simulink model "MVB4Single"  (R2013b)
settings: Solver=FixedStepDiscrete  SolverMode=SingleTasking  StartTime=0  StopTime=8000  RelTol=1e-3
model workspace (MAT data in the model file):
  logicAddr = 2
settings Model: Creator=qiji  LastModifiedBy=qiji
settings DataIOCC: SignalLoggingSaveFormat=ModelDataLogs
settings OptimizationCC: BlockReduction=off  ConditionallyExecuteInputs=off  InlineParams=on
settings DebuggingCC: UnderspecifiedInitializationDetection=Simplified  MultiTaskDSMMsg=warning  MultiTaskCondExecSysMsg=none  SingleTaskRateTransMsg=error  SFUnusedDataAndEventsDiag=none
settings RTWCC: IncludeERTFirstTime=on
settings GRTTargetCC: CodeReplacementLibrary=None  CPPClassGenCompliant=on
settings ConfigurationSet: Description=SimMechanics 2G

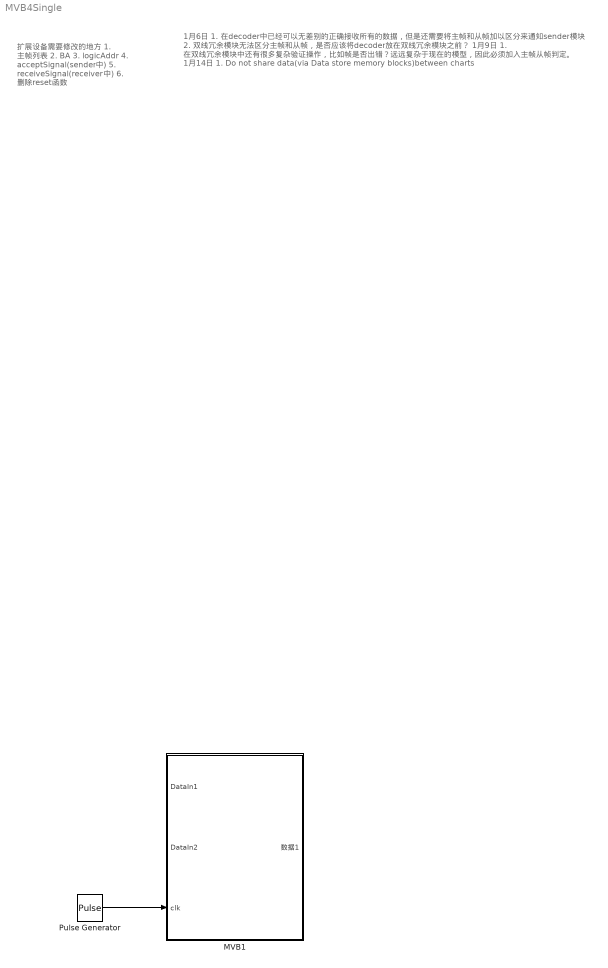
== system MVB4Single ==
  note: 扩展设备需要修改的地方
      | 1. 主帧列表
      | 2. BA
      | 3. logicAddr
      | 4. acceptSignal(sender中)
      | 5. receiveSignal(receiver中)
      | 6. 删除reset函数
  note: 1月6日
      | 1. 在decoder中已经可以无差别的正确接收所有的数据，但是还需要将主帧和从帧加以区分来通知sender模块
      | 2. 双线冗余模块无法区分主帧和从帧，是否应该将decoder放在双线冗余模块之前？
      | 1月9日
      | 1. 在双线冗余模块中还有很多复杂验证操作，比如帧是否出错？远远复杂于现在的模型，因此必须加入主帧从帧判定。
      | 1月14日
      | 1. Do not share data(via Data store memory blocks)between charts
  MVB1 : Subsystem
  Pulse Generator : DiscretePulseGenerator  Amplitude=true
  wires:
  Pulse Generator/1 -> MVB1/3("clk ")

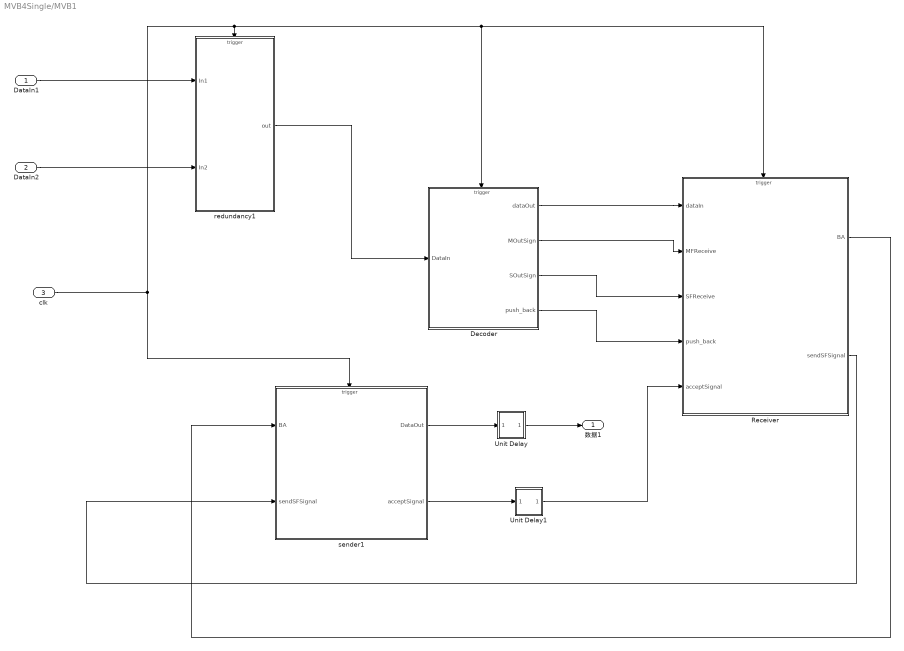
== system MVB4Single/MVB1 ==
  DataIn1 : Inport
  DataIn2 : Inport  Port=2
  "clk " : Inport  Port=3
  Decoder : Stateflow chart  TreatAsAtomicUnit=on
  Receiver : Stateflow chart  TreatAsAtomicUnit=on
  Unit Delay : Subsystem
  Unit Delay1 : Subsystem
  redundancy1 : Stateflow chart  TreatAsAtomicUnit=on
  sender1 : Stateflow chart  TreatAsAtomicUnit=on
  数据1 : Outport
  wires:
  DataIn1/1 -> redundancy1/1(In1)
  DataIn2/1 -> redundancy1/2(In2)
  redundancy1/1(out) -> Decoder/1(DataIn)
  Unit Delay/1(Out) -> 数据1/1
  "clk "/1 -> Decoder/Trigger, Receiver/Trigger, redundancy1/Trigger, sender1/Trigger
  Decoder/1(dataOut) -> Receiver/1(dataIn)
  Decoder/2(MOutSign) -> Receiver/2(MFReceive)
  Decoder/3(SOutSign) -> Receiver/3(SFReceive)
  Decoder/4(push_back) -> Receiver/4(push_back)
  Receiver/1(BA) -> sender1/1(BA)
  Unit Delay1/1(Out) -> Receiver/5(acceptSignal)
  Receiver/2(sendSFSignal) -> sender1/2(sendSFSignal)
  sender1/1(DataOut) -> Unit Delay/1(In1)
  sender1/2(acceptSignal) -> Unit Delay1/1(In1)

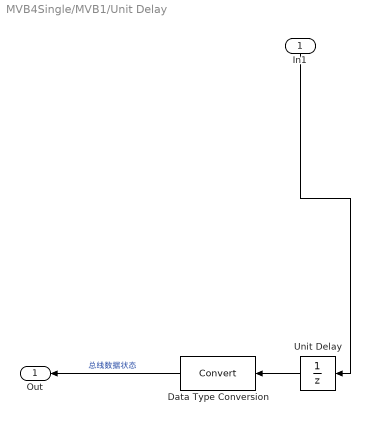
== system MVB4Single/MVB1/Unit Delay ==
  In1 : Inport
  Data Type Conversion : DataTypeConversion
  Unit Delay : UnitDelay  SampleTime=-1
  Out : Outport
  wires:
  In1/1 -> Unit Delay/1
  Unit Delay/1 -> Data Type Conversion/1
  Data Type Conversion/1 -> Out/1  "总线数据状态"

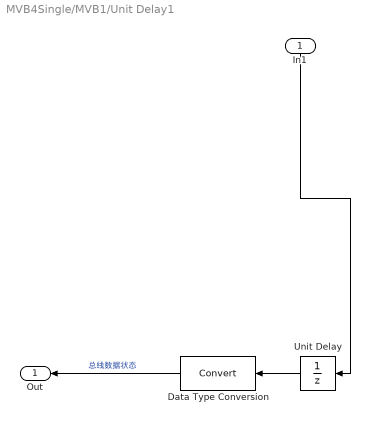
== system MVB4Single/MVB1/Unit Delay1 ==
  In1 : Inport
  Data Type Conversion : DataTypeConversion
  Unit Delay : UnitDelay  SampleTime=-1
  Out : Outport
  wires:
  Data Type Conversion/1 -> Out/1  "总线数据状态"
  Unit Delay/1 -> Data Type Conversion/1
  In1/1 -> Unit Delay/1

== stateflow chart MVB4Single/MVB1/redundancy1 ==
  settings: executeAtInitialization=1  initializeOutput=1
  state sign_maker [parallel]
    settings: executionOrder=1
    state sign1 [parallel]
      settings: executionOrder=1
      state trans
        sign_maker.sign1.trans -> sign_maker.sign1.trans [order 1] : CLK
            | {
            | buffer = bitoperate.shiftbit(buffer, 1) + In1;
            | count++;
            | }
      state none
        en:
        count=2;
        buffer=1;
      state judge
      (default) -> sign_maker.sign1.none : {count=0;buffer=0;}
      sign_maker.sign1.none -> sign_maker.sign1.trans : [In1==1]{sign1 = true;}
      sign_maker.sign1.judge -> sign_maker.sign1.trans [order 2] : {buffer=0;count=0;}
      sign_maker.sign1.judge -> sign_maker.sign1.none [order 1] : [judgeEnd(buffer)]
          | {sign1 = false;}
      sign_maker.sign1.trans -> sign_maker.sign1.judge [order 1] : [count==32]
          | {buffer=ManchesterDecoding(buffer);
          | }
    state sign2 [parallel]
      settings: executionOrder=2
      state trans
        sign_maker.sign2.trans -> sign_maker.sign2.trans [order 1] : CLK
            | {
            | buffer = bitoperate.shiftbit(buffer, 1) + In2;
            | count++;
            | }
      state none
        en:
        count=2;
        buffer=1;
      state judge
      (default) -> sign_maker.sign2.none : {count=0;buffer=0;}
      sign_maker.sign2.none -> sign_maker.sign2.trans : [In2==1]{sign2 = true;}
      sign_maker.sign2.judge -> sign_maker.sign2.trans [order 2] : {buffer=0;count=0;}
      sign_maker.sign2.judge -> sign_maker.sign2.none [order 1] : [judgeEnd(buffer)]
          | {sign2 = false;}
      sign_maker.sign2.trans -> sign_maker.sign2.judge [order 1] : [count==32]
          | {buffer=ManchesterDecoding(buffer);
          | }
  state bitoperate [group]
  note: 从上一个接收事件后总线寂静1.4ms则产生一总线寂静的通知
  state Timer1 [parallel]
    settings: executionOrder=2
    state Timer
    state start
    state TimeOut
      entry:
      trust = false;
    start -> Timer : [judge(sign1, sign2, trust) == false]
    (default) -> start
    Timer -> start [order 1] : [judge(sign1, sign2,  trust) == true]
    TimeOut -> start
    Timer -> TimeOut [order 2] : [after(140, CLK) && judge(sign1, sign2,  trust) == false]
  note: 上一个主帧接收后1.3ms没有收到主帧产生一个主帧超时的通知。
  note: 收到主帧后42.7us没有收到从帧产生从帧超时的通知。
  note: 信任线未收到数据，而观察线收到数据时切换
  state observer [parallel]
    settings: executionOrder=3
    state A
      entry:
      trust = true;
    state B
      entry:
      trust = false;
    observer.A -> observer.B : [judge(sign1, sign2, trust) == false]
    (default) -> observer.A
    observer.B -> observer.A : [judge(sign1, sign2, trust) == false]
  state trans [parallel]
    settings: executionOrder=4
    state A
      during:
      out = In1;
    state B
      during:
      out = In2;
    trans.A -> trans.B : [trust == false]{out = In2;}
    (default) -> trans.A
    trans.B -> trans.A : [trust == true]{out = In1;}
  data: r function_output boolean; data function_input uint16; buffer local uint32; count local uint32; buffer local uint32; count local uint32; r function_output uint32; data function_input uint32; num function_input uint32; r function_output uint32; data function_input uint32; num function_input uint32; r function_output uint32; r function_output boolean; dataIn1 function_input uint32; dataIn2 function_input uint32; t function_input boolean; r function_output boolean; dataIn1 function_input boolean; dataIn2 function_input boolean; t function_input boolean; In1 input uint32; In2 input uint32; out output uint32; trust local boolean =true; sign1 local boolean; sign2 local boolean
  events: CLK input RISING_EDGE_EVENT
  function r = judgeEnd(data):
    | function r = judgeEnd(data)
    | bit1 = bitget(data, 1);
    | bit2 = bitget(data, 2);
    | bit3 = bitget(data, 3);
    | bit4 = bitget(data, 4);
    | if bit1==1 && bit2==1 && bit3==0 && bit4==0
    |     r = true;
    | else
    |     r = false;
    | end
  function r = ManchesterDecoding(data):
    | function r = ManchesterDecoding(data)
    | r = uint32(0);
    | for i = (1:2:32)
    |     x0 = bitget(data, i);
    |     x1 = bitget(data, i+1);
    |     if x0==0 && x1==1
    |         r = bitset(r, (i+1)/2, 1);
    |     else
    |         r = bitset(r, (i+1)/2, 0);
    |     end
    | end
  function r = getbit(num):
    | function r = getbit(num)
    | r = bitget(num, 32);
  function r = shiftbit(data, num):
    | function r = shiftbit(data, num)
    | r = bitshift(data, num);
    | %for i=1:cnt
    | %   r = bitset(r, i, 0);
    | %end
  function r = judge(dataIn1, dataIn2, t):
    | function r = judge(dataIn1, dataIn2, t)
    | r = true;
    | if t == true
    |     if dataIn1==false
    |         r = false;
    |     end
    | else
    |     if dataIn2==false
    |         r = false;
    |     end
    | end
  function r = judge( dataIn1, dataIn2, t):
    | function r = judge( dataIn1, dataIn2, t)
    | r = true;
    | % 如果数据线1没有收到数据而数据线2收到了
    | if t == true
    |     if dataIn1==false && dataIn2==true
    |         r = false;
    |     end
    | else
    |     if dataIn2==false && dataIn1==true
    |         r = false;
    |     end
    | end

== stateflow chart MVB4Single/MVB1/sender1 ==
  settings: executeAtInitialization=1  initializeOutput=1
  state SFSender [parallel]
    settings: executionOrder=1
    note: send**Signd的置位在接收到了请求数据的主帧后置位
    state sender [parallel]
      settings: executionOrder=1
      state wait
      state sendRandomSF
      state sendOK
      state sendInfo
      state transmission
        en:
        enterTrans = true;
        ex:
        enterTrans = false;
      (default) -> SFSender.sender.wait
      SFSender.sender.wait -> sendRandomSF [order 1] : [sendSFSignal==1]
      SFSender.sender.wait -> sendInfo [order 3] : [ sendSFSignal==2]
      SFSender.sender.wait -> sendOK [order 2] : [sendSFSignal==3]
      sendRandomSF -> SFSender.sender.transmission : {SFIndex = uint8(0);}
      sendOK -> SFSender.sender.transmission : {SFIndex = uint8(2);
          | init();
          | }
      sendInfo -> SFSender.sender.transmission : {SFIndex = uint8(1);}
      SFSender.sender.transmission -> SFSender.sender : [SFTransDone == true]
          | {DataOut = uint32(0);}
          | /{SFTransDone = false;}
    state sendHolder [parallel]
      settings: executionOrder=2
      state judge
      state full
        SFSender.sendHolder.full -> SFSender.sendHolder.full [order 1] : CLK
            | {
            | DataOut = bitoperate.getbit(input);
            | input = bitoperate.shiftbit(input, uint32(1));
            | count = count + uint8(1);
            | }
      state empty
      SFSender.sendHolder.judge -> SFSender.sendHolder.empty [order 2] : {
          | SFCurrentIndex = uint8(2);
          | SFTransDone = true;
          | }
      SFSender.sendHolder.full -> SFSender.sendHolder.judge [order 1] : [count == uint8(32)]
          | {
          | SFCurrentIndex = SFCurrentIndex + uint8(1);
          | }
      SFSender.sendHolder.judge -> SFSender.sendHolder.full [order 1] : [SFCurrentIndex <= SFT[SFIndex*16 + 1]]
          | {
          | input = ManchesterEncoding(uint32(SFT[SFIndex*16+SFCurrentIndex]));
          | count = uint8(0);
          | }
      (default) -> SFSender.sendHolder.empty : {
          | SFCurrentIndex = uint8(2);
          | SFTransDone = false;
          | }
      SFSender.sendHolder.empty -> SFSender.sendHolder.full : [enterTrans == true]
          | {
          | input = ManchesterEncoding(uint32(SFT[SFIndex*16+SFCurrentIndex]));
          | DataOut = uint32(0);
          | count = uint8(0);
          | }
  state MFSender [parallel]
    settings: executionOrder=2
    state sender [parallel]
      settings: executionOrder=2
      state transmission
        en:
        enterTrans = true;
        acceptSignal =setAcceptSignal(MFT[MFIndex*16+3]);
        ex:
        enterTrans = false;
      state sleep
      state wait
      (default) -> sleep : {
          | init();
          | }
      MFSender.sender.transmission -> sleep : [MFTransDone==true]
          | {
          | DataOut = uint32(0);
          | MFIndex = MFIndex + uint8(1);
          | MFTransDone=false;
          | }
      sleep -> MFSender.sender.wait : every(150, CLK)
          | [master==true]
      MFSender.sender.wait -> MFSender.sender.transmission
    state sendHolder [parallel]
      settings: executionOrder=3
      state judge
      state full
        MFSender.sendHolder.full -> MFSender.sendHolder.full [order 1] : CLK
            | {
            | DataOut = bitoperate.getbit(input);
            | input = bitoperate.shiftbit(input, uint32(1));
            | count = count + uint8(1);
            | }
      state empty
      MFSender.sendHolder.judge -> MFSender.sendHolder.empty [order 2] : {
          | MFCurrentIndex = uint8(2);
          | MFTransDone=true;
          | }
      MFSender.sendHolder.full -> MFSender.sendHolder.judge [order 1] : [count == uint8(32)]
          | {
          | MFCurrentIndex = MFCurrentIndex + uint8(1);
          | }
      MFSender.sendHolder.judge -> MFSender.sendHolder.full [order 1] : [MFCurrentIndex <= MFT[MFIndex*16 + 1]]
          | {
          | input =ManchesterEncoding(uint32(MFT[MFIndex*16+MFCurrentIndex]));
          | count = uint8(0);
          | }
      (default) -> MFSender.sendHolder.empty : {
          | MFCurrentIndex = uint8(2);
          | MFTransDone=false;
          | }
      MFSender.sendHolder.empty -> MFSender.sendHolder.full : [enterTrans == true]
          | {
          | input = ManchesterEncoding(uint32(MFT[MFIndex*16+MFCurrentIndex]));
          | DataOut = uint32(0);
          | count = uint8(0);
          | }
    state BAHolder [parallel]
      settings: executionOrder=1
      state false
        du:
        master = false;
      state true
        du:
        master = true;
      false -> true : [BA == true]
          | {master = true;}
      (default) -> true
      true -> false : [BA == true]
          | {master =false;}
  state init [function]
    note: F_code=0
        | addr=2
        | 0010//1100/0111/0001
        | 0101//0000/0000/0000
        | 0010//1010/1000/1110
        | 0000/0000/0011//0011
        | F_code=8
        | addr=2
        | 0010//1100/0111/0001
        | 0101//1000/0000/0000
        | 0010//1010/1000/1110
        | 0000/0000/0011//0011
        | F_code=0
        | addr=2
        | 0010//1100/0111/0001
        | 0101//1111/0000/0000
        | 0010//1010/1000/1110
        | 0000/0000/0011//0011
    note: 请求随机从帧
        | 请求随机从帧
        | 请求2号的信息
        | 请求转移到2号
    note: SFT(1)代表随机的从帧
        | SFT(2)代表回复接受主权
        | SFT(3)代表回复设备ACT和BA
    (default) -> (junction 77) : {
        | MFIndex = uint8(0);
        | acceptSignal = uint8(0);
        | MFT[1] = uint16(5);
        | MFT[2] = uint16(11377);
        | MFT[3] = uint16(20480);
        | MFT[4] = uint16(10894);
        | MFT[5] = uint16(51);
        |
        | MFT[17] = uint16(5);
        | MFT[18] = uint16(11377);
        | MFT[19] = uint16(20480);
        | MFT[20] = uint16(14990);
        | MFT[21] = uint16(51);
        |
        | MFT[33] = uint16(5);
        | MFT[34] = uint16(11377);
        | MFT[35] = uint16(22528);
        | MFT[36] = uint16(10894);
        | MFT[37] = uint16(51);
        |
        | MFT[49] = uint16(5);
        | MFT[50] = uint16(11377);
        | MFT[51] = uint16(24320);
        | MFT[52] = uint16(10894);
        | MFT[53] = uint16(51);
        |
        |
        | SFT[1] = uint16(4);
        | SFT[2] = uint16(10894);
        | SFT[3] = uint16(12428);
        | SFT[4] = uint16(19);
        | SFT[17] = uint16(4);
        | SFT[18] = uint16(10894);
        | SFT[19] = uint16(12832);
        | SFT[20] = uint16(3);
        | SFT[33] = uint16(4);
        | SFT[34] = uint16(10894);
        | SFT[35] = uint16(14464);
        | SFT[36] = uint16(3);
        | }
  state bitoperate [group]
  note: MFT(1) = 5;
      | MFT(2) = 11377;
      | MFT(3) = 20480;
      | MFT(4) = 10894;
      | MFT(5) = 51;
      |
      | MFT(17) = 5;
      | MFT(18) = 11377;
      | MFT(19) = 20480;
      | MFT(20) = 10894;
      | MFT(21) = 51;
      |
      | MFT(33) = 5;
      | MFT(34) = 11377;
      | MFT(35) = 22528;
      | MFT(36) = 10894;
      | MFT(37) = 51;
      |
      | MFT(49) = 5
      | MFT(50) = 11377;
      | MFT(52) = 24320;
      | MFT(53) = 10894;
      | MFT(54) = 51;
  data: SFCurrentIndex local uint8; count local uint8; input local uint32; SFTransDone local boolean; SFIndex local uint8; enterTrans local boolean; data function_input uint16; Signal function_output uint8; bit1 temporary uint16; bit2 temporary uint16; bit3 temporary uint16; bit0 temporary uint16; i function_input double; r function_output uint8; MFCurrentIndex local uint8; count local uint8; input local uint32; MFTransDone local boolean; enterTrans local boolean; data function_input uint32; r function_output uint32; r function_output uint32; data function_input uint32; num function_input uint32; r function_output uint32; data function_input uint32; num function_input uint32; r function_output uint32; BA input boolean; sendSFSignal input uint8; MFT local uint16 size=100; SFT local uint16 size=100; DataOut output uint32; acceptSignal output uint8; MFIndex local uint8; master local boolean
  events: CLK input RISING_EDGE_EVENT
  function Signal = setAcceptSignal(data):
    | function Signal = setAcceptSignal(data)
    | bit0 = uint16(bitget(data, 9));
    | bit1 = uint16(bitget(data, 10));
    | bit2 = uint16(bitget(data, 11));
    | bit3 = uint16(bitget(data, 12));
    | fcode = bit0+bit1*2+bit2*4+bit3*8;
    | Signal=uint8(0);
    | if fcode==0
    |     Signal=uint8(1);
    | elseif fcode==8
    |     Signal=uint8(2);
    | elseif fcode==15
    |     Signal=uint8(3);
    | end
  function r = reset(i):
    | function r = reset(i)
    | if i==2
    |     r = uint8(0);
    | else
    |     r = uint8(i);
    | end
  function r = ManchesterEncoding(data):
    | function r = ManchesterEncoding(data)
    | r = data;
    | for i = 1:16
    |     x = bitget(data, i);
    |     if x == 0
    |         r = bitset(r, i*2-1, 1);
    |         r = bitset(r, i*2, 0);
    |     else
    |         r = bitset(r, i*2-1, 0);
    |         r = bitset(r, i*2, 1);
    |     end
    | end
  function r = ManchesterDecoding(data):
    | function r = ManchesterDecoding(data)
    | r = uint32(0);
    | for i = (1:2:32)
    |     x0 = bitget(data, i);
    |     x1 = bitget(data, i+1);
    |     if x0==0 && x1==1
    |         r = bitset(r, (i+1)/2, 1);
    |     else
    |         r = bitset(r, (i+1)/2, 0);
    |     end
    | end
  function r = getbit(num):
    | function r = getbit(num)
    | r = bitget(num, 32);
  function r = shiftbit(data, num):
    | function r = shiftbit(data, num)
    | r = bitshift(data, num);
    | %for i=1:cnt
    | %   r = bitset(r, i, 0);
    | %end

== stateflow chart MVB4Single/MVB1/Receiver ==
  settings: sampleTime=4.1666666667e-8  executeAtInitialization=1  initializeOutput=1
  state receiveMF [parallel]
    settings: executionOrder=1
    state wait
      en:
      [buffer, BufferIndex]= initBuffer();
    state wait4MFEnd
    state judgeAddr
    state MFReceive
    state MFcode0
    state MFcode8
    state MFcode15
    state MTrans
    note: 如果收到了f_code为15的主帧，则应该获得主权
    (default) -> receiveMF.wait
    judgeAddr -> receiveMF.wait [order 2]
    MTrans -> receiveMF.wait
    receiveMF.wait -> wait4MFEnd : [MFReceive==true]
    wait4MFEnd -> judgeAddr : [MFReceive == false]
        | {fcodeIn = uint8(getFCode(buffer));
        | addrIn = uint16(getAddr(buffer));
        | }
    judgeAddr -> MFReceive [order 1] : [addrIn == LogicAddr]
    MFReceive -> MFcode0 [order 2] : [fcodeIn == 0]
    MFReceive -> MFcode8 [order 3] : [fcodeIn == 8]
    MFReceive -> MFcode15 [order 1] : [fcodeIn == 15 ]
    MFcode0 -> MTrans : {sendSFSignal=1;}
    MFcode8 -> MTrans : {sendSFSignal=2;}
    MFcode15 -> MTrans : {sendSFSignal=3;
        | BAPrepare = true;}
  state receiveSF1 [parallel]
    settings: executionOrder=3
    note: acceptSF, acceptACT, acceptDomain在发送完主帧以后，根据主帧的类型进行相应的置位
        | 收到fcode为8的从帧之后，说明目标设备已经返回了OK，这时应该将BA置位
    state wait
      en:
      initBuffer();
      temp=0;
    state wait4SF
    state wait4ACT
    state wait4Domain
    state wait4SFEnd
    state test
    state STrans
    (default) -> receiveSF1.wait
    (junction 287) -> receiveSF1.wait : {
        | BufferIndex = 0;
        | }
    receiveSF1.wait -> (junction 287) [order 4] : [SFReceive == true]
        | {BA = getBA(BAPrepare)
        | BAPrepare = false;}
    receiveSF1.wait -> wait4SF [order 1] : [acceptSignal == 1]
        | {
        | temp=1;
        | }
    receiveSF1.wait -> wait4ACT [order 2] : [acceptSignal==2]
        | {
        | temp=2;
        | }
    receiveSF1.wait -> wait4Domain [order 3] : [acceptSignal==3]
        | {
        | temp=3;
        | }
    wait4SF -> wait4SFEnd : [SFReceive == true]
    wait4ACT -> wait4SFEnd : [SFReceive==true]
    wait4Domain -> wait4SFEnd : [SFReceive==true]
    test -> (junction 287) [order 2]
    STrans -> (junction 287) : [SFReceive == false]
        | {
        | BA = reset(temp);
        | }
    wait4SFEnd -> test : [SFReceive == false]
    test -> STrans [order 1] : [judge(temp, buffer)]
  state Buffer [parallel]
    settings: executionOrder=2
    state wait
    state push_back
      en:
      buffer[BufferIndex]=dataIn;
      BufferIndex = BufferIndex+1;
    (default) -> Buffer.wait : {
        | BufferIndex = uint8(0);
        | }
    Buffer.wait -> push_back : [push_back==1]
    push_back -> Buffer.wait
  data: tmp function_input uint8; r function_output boolean; prepare function_input boolean; r function_output boolean; tmp function_input uint8; data function_input uint16 size=16; r function_output boolean; temp local uint8; r function_output uint16 size=16; index function_output uint8; data function_input uint32; num function_input uint32; r function_output uint32; data function_input uint16 size=16; r function_output uint16; bit1 temporary uint16; bit2 temporary uint16; bit3 temporary uint16; bit0 temporary uint16; data function_input uint32; r function_output uint32; r function_output uint32; data function_input uint32; data function_input uint16 size=16; r function_output uint16; dataIn input uint32; MFReceive input boolean; SFReceive input boolean; fcodeIn local uint8; addrIn local uint16; BA output boolean; BufferIndex local uint8; buffer local uint16 size=16 =[0,0,0,0,0,0,0,0,0,0,0,0,0,0,0,0]; push_back input boolean; LogicAddr constant uint8 =1; sendSFSignal output uint8 =0; acceptSignal input uint8; BAPrepare local boolean
  events: CLK input RISING_EDGE_EVENT
  function r = reset(tmp):
    | function r = reset(tmp)
    | r = false;
    | if tmp==3
    |     r = true;
    | end;
  function r = getBA(prepare):
    | function r = getBA(prepare)
    | r = false;
    | if prepare == true
    |     r = true;
    | end;
  function r = judge(tmp, data):
    | function r = judge(tmp, data)
    | if tmp==1
    |     r = true;
    | elseif tmp==2 && bitget(data(2), 6)
    |     r = true;
    | elseif tmp==3 && bitget(data(2), 8)
    |     r = true;
    | else
    |     r = false;
    | end
  function [r, index] = initBuffer:
    | function [r, index] = initBuffer
    | r = [(uint16(0));(uint16(0));(uint16(0));(uint16(0));...
    |     (uint16(0));(uint16(0));(uint16(0));(uint16(0));...
    |     (uint16(0));(uint16(0));(uint16(0));(uint16(0));...
    |     (uint16(0));(uint16(0));(uint16(0));(uint16(0))];
    | index=uint8(0);
  function r = getbit(data, num):
    | function r = getbit(data, num)
    | r = bitget(uint32(data), num);
  function r = getFCode(data):
    | function r = getFCode(data)
    | bit0 = bitget(data(2), 9);
    | bit1 = bitget(data(2), 10);
    | bit2 = bitget(data(2), 11);
    | bit3 = bitget(data(2), 12);
    | r = bit0+bit1*2+bit2*4+bit3*8;
  function r = ManchesterEncoding(data):
    | function r = ManchesterEncoding(data)
    | r = data;
    | for i = 1:16
    |     x = bitget(data, i);
    |     if x == 0
    |         r = bitset(r, i*2-1, 1);
    |         r = bitset(r, i*2, 0);
    |     else
    |         r = bitset(r, i*2-1, 0);
    |         r = bitset(r, i*2, 1);
    |     end
    | end
  function r = ManchesterDecoding(data):
    | function r = ManchesterDecoding(data)
    | r = uint32(0);
    | for i = (1:2:32)
    |     x0 = bitget(data, i);
    |     x1 = bitget(data, i+1);
    |     if x0==0 && x1==1
    |         r = bitset(r, (i+1)/2, 1);
    |     else
    |         r = bitset(r, (i+1)/2, 0);
    |     end
    | end
  function r = getAddr(data):
    | function r = getAddr(data)
    | %取出buffer(2)后8位
    | high8 = bitshift(bitshift(uint16(data(2)), 8), -4);
    | % 取出buffer(3)前4位
    | low4 = bitshift(uint16(data(3)), -12);
    | r = high8 + low4;

== stateflow chart MVB4Single/MVB1/Decoder ==
  settings: executeAtInitialization=1  initializeOutput=1
  state judge_data [parallel]
    settings: executionOrder=1
    state MF
      en:
      MOutSign= true;
    state wait4Data
      en:
      [buffer, index] = initBuffer();
    state judgeData
      en:
      receive_complete = false;
    state end
    state SF
      en:
      SOutSign=true;
    judgeData -> MF [order 1] : [judge(buffer)==1]
    MF -> end
    wait4Data -> judgeData : [receive_complete == true]
    (default) -> wait4Data
    judgeData -> wait4Data [order 3] : [judge(buffer)==0]
    judgeData -> SF [order 2] : [judge(buffer)==2]
    end -> wait4Data
    SF -> end
  note: 0010//1100/0111/0001
      | 0101//0000/0000/0000
      | 0001//1010/1000/1110
      | 0000/0000/0011//0011
  state receiver [parallel]
    settings: executionOrder=2
    state decodeSF
      decodeSF -> decodeSF [order 1] : CLK
          | {
          | ans = bitoperate.shiftbit(ans, 1) + DataIn;
          | count++;
          | }
    note: 首先接受所有的数据，当接受完毕以后，再通知另外一个子系统判断
        | 从帧和主帧，并对dataout赋值。
    state judge
      en:
      ans = 0;
    state start
    decodeSF -> judge [order 1] : [count==32]
        | {
        | buffer[index] = ManchesterDecoding(ans);
        | count=0;
        | dataOut = buffer[index];
        | push_back = 1;
        | }
    start -> decodeSF : [DataIn == 1]
        | {
        | count = 2;
        | ans=1;
        | }
    judge -> decodeSF [order 1] : [!judgeEnd(buffer[index])]
        | {index++;}
    judge -> start [order 2] : {
        | receive_complete = true;
        | dataOut = 0;
        | }
    (default) -> start
  state bitoperate [group]
  data: r function_output double; dataBuffer function_input uint16 size=16; r function_output boolean; data function_input uint16; num function_input uint32; r function_output uint32; data function_input uint32; num function_input uint32; r function_output uint32; r function_output uint16 size=16; i function_output uint8; r function_output uint32; data function_input uint32; DataIn input uint32; dataOut output uint32; count local uint32; MOutSign output boolean; SOutSign output boolean; ans local uint32; buffer local uint16 size=16; index local uint8; push_back output boolean; receive_complete local boolean =false
  events: CLK input RISING_EDGE_EVENT
  function r = judge(dataBuffer):
    | function r = judge(dataBuffer)
    | low12 = bitshift(dataBuffer(1), 4);
    | high4 = bitshift(dataBuffer(2), -12);
    | start = low12 + high4;
    | r = 0;
    | if start == 50965
    |     r = 1;
    | elseif start == 43235
    |     r = 2;
    | end
  function r = judgeEnd(data):
    | function r = judgeEnd(data)
    | bit1 = bitget(data, 1);
    | bit2 = bitget(data, 2);
    | bit3 = bitget(data, 3);
    | bit4 = bitget(data, 4);
    | if bit1==1 && bit2==1 && bit3==0 && bit4==0
    |     r = true;
    | else
    |     r = false;
    | end
  function r = getbit(num):
    | function r = getbit(num)
    | r = bitget(num, 32);
  function r = shiftbit(data, num):
    | function r = shiftbit(data, num)
    | r = bitshift(data, num);
    | %for i=1:cnt
    | %   r = bitset(r, i, 0);
    | %end
  function [r, i] = initBuffer:
    | function [r, i] = initBuffer
    | r = [(uint16(0));(uint16(0));(uint16(0));(uint16(0));...
    |     (uint16(0));(uint16(0));(uint16(0));(uint16(0));...
    |     (uint16(0));(uint16(0));(uint16(0));(uint16(0));...
    |     (uint16(0));(uint16(0));(uint16(0));(uint16(0))];
    | i=uint8(0);
  function r = ManchesterDecoding(data):
    | function r = ManchesterDecoding(data)
    | r = uint32(0);
    | for i = (1:2:32)
    |     x0 = bitget(data, i);
    |     x1 = bitget(data, i+1);
    |     if x0==0 && x1==1
    |         r = bitset(r, (i+1)/2, 1);
    |     else
    |         r = bitset(r, (i+1)/2, 0);
    |     end
    | end
